simulink model "fz7_7"  (R2014a)
settings: Solver=ode45  StartTime=0.0  StopTime=50000  RelTol=1e-3
values from neighbouring files (symbols this model uses):
  SymbolRate = 1000    [eg7_11.m]    (also in eg7_2.m = 2; eg7_4.m = 2; eg7_7.m = 2)
libraries: commutil2 x4, commsink2 x2, commdigbbndpm3 x2, commchan3 x1, commrandsrc2 x1
settings Model: Creator=tzb  LastModifiedBy=tzb
settings DebuggingCC: SolverPrmCheckMsg=none

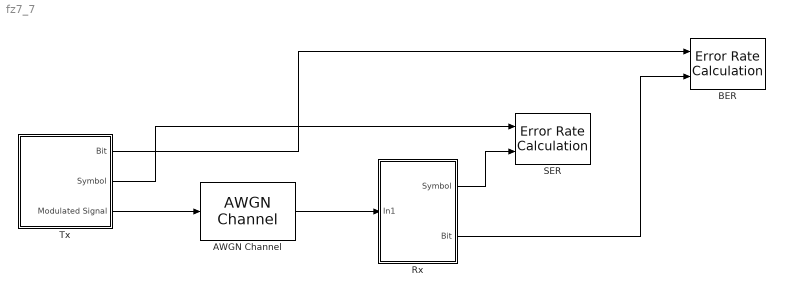
== system fz7_7 ==
  AWGN Channel : commchan3/AWGN Channel  InputProcessing=Columns as channels (frame based)  seed=67  noiseMode="Signal to noise ratio  (Es/No)"  EbNodB=10  EsNodB=SNR  SNRdB=10  bitsPerSym=1  Ps=1  Tsym=1/SymbolRate  variance=1
  BER : commsink2/Error Rate Calculation  N=0  st_delay=0  cp_mode=Entire frame  subframe=[]  PMode=Workspace  WsName=BER  RsMode2=off  stop=off  numErr=100  maxBits=1e6
  Rx : Subsystem
  SER : commsink2/Error Rate Calculation  N=0  st_delay=0  cp_mode=Entire frame  subframe=[]  PMode=Workspace  WsName=SER  RsMode2=off  stop=off  numErr=100  maxBits=1e6
  Tx : Subsystem
  wires:
  Tx/3(Modulated Signal) -> AWGN Channel/1
  AWGN Channel/1 -> Rx/1(In1)
  Rx/1(Symbol) -> SER/2
  Rx/2(Bit) -> BER/2
  Tx/1(Bit) -> BER/1
  Tx/2(Symbol) -> SER/1

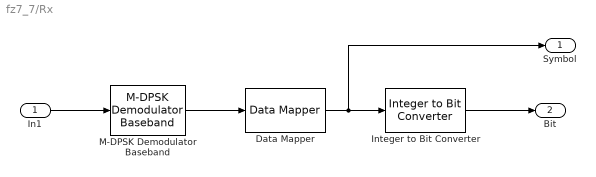
== system fz7_7/Rx ==
  In1 : Inport
  Data Mapper : commutil2/Data Mapper  MapMode=Gray to Binary  M=4  MapVec=[0 1 3 2 7 6 4 5]
  Integer to Bit Converter : commutil2/Integer to Bit Converter  nbits=2  signedInputValues=Unsigned  bitOrder=MSB first  outDtype=Inherit via internal rule
  M-DPSK Demodulator Baseband : commdigbbndpm3/M-DPSK Demodulator Baseband  M=4  OutType=Integer  Dec=Gray  Ph=pi/8  outDtype1=Inherit via internal rule  outDtype2=Inherit via internal rule
  Symbol : Outport
  Bit : Outport  Port=2
  wires:
  In1/1 -> M-DPSK Demodulator Baseband/1
  Data Mapper/1 -> Symbol/1, Integer to Bit Converter/1
  M-DPSK Demodulator Baseband/1 -> Data Mapper/1
  Integer to Bit Converter/1 -> Bit/1

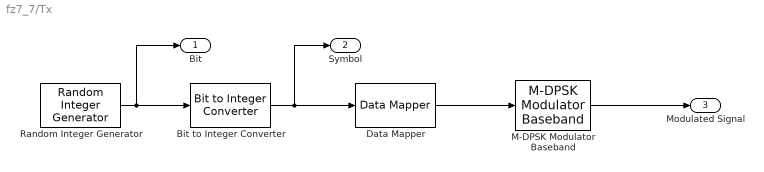
== system fz7_7/Tx ==
  Bit to Integer Converter : commutil2/Bit to Integer Converter  nbits=2  bitOrder=MSB first  signedOutputValues=Unsigned  outDtype=Inherit via internal rule  outDtypeSigned=Inherit via internal rule
  Data Mapper : commutil2/Data Mapper  MapMode=Binary to Gray  M=4  MapVec=[0 1 3 2 7 6 4 5]
  M-DPSK Modulator Baseband : commdigbbndpm3/M-DPSK Modulator Baseband  M=4  InType=Integer  Enc=Gray  Ph=pi/8  outDtype=double
  Random Integer Generator : commrandsrc2/Random Integer Generator  mul=2  seed=37  Ts=1/(2*SymbolRate)  frameBased=on  sampPerFrame=2*SymbolRate  orient=off  outDataType=double
  Bit : Outport
  Symbol : Outport  Port=2
  Modulated Signal : Outport  Port=3
  wires:
  M-DPSK Modulator Baseband/1 -> Modulated Signal/1
  Random Integer Generator/1 -> Bit/1, Bit to Integer Converter/1
  Bit to Integer Converter/1 -> Symbol/1, Data Mapper/1
  Data Mapper/1 -> M-DPSK Modulator Baseband/1
